simulink model "simulation_pdy_pdx_theta_discreteV2"  (R2015a)
settings: Solver=ode45  StartTime=0.0  StopTime=8000.0  RelTol=1e-3
libraries: simulink x1
settings Model: Creator=MateusVendramini  LastModifiedBy=MateusVendramini
settings SolverCC: AlgebraicLoopSolver=LineSearch

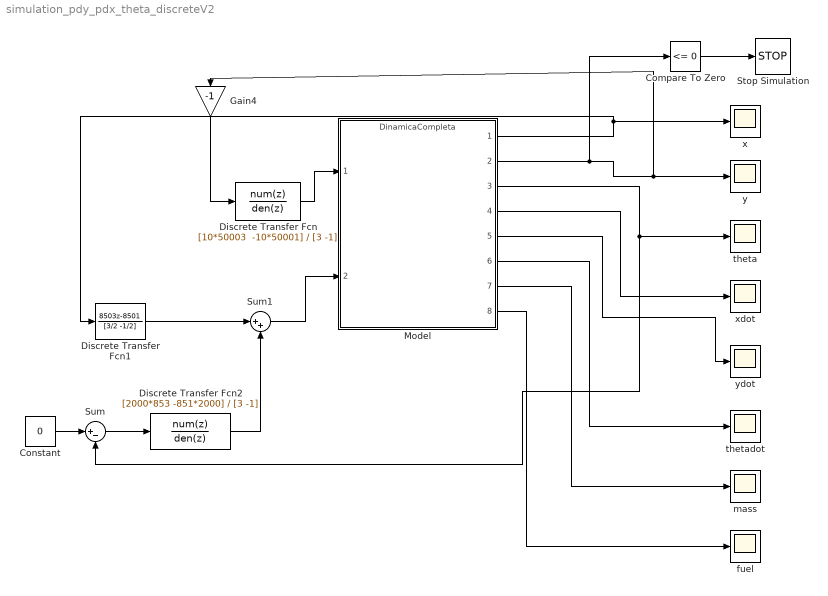
== system simulation_pdy_pdx_theta_discreteV2 ==
  Compare To Zero : simulink/Logic and Bit Operations/Compare To Zero  relop=<=  OutDataTypeStr=boolean
  Constant : Constant  Value=0
  Discrete Transfer Fcn : DiscreteTransferFcn  Numerator="[10*50003  -10*50001]"  Denominator=[3 -1]  SampleTime=0.01
  Discrete Transfer Fcn1 : DiscreteTransferFcn  Numerator=[8503 -8501]  Denominator=[3/2 -1/2]  SampleTime=0.01
  Discrete Transfer Fcn2 : DiscreteTransferFcn  Numerator=[2000*853 -851*2000]  Denominator=[3 -1]  SampleTime=0.01
  Gain4 : Gain  Gain=-1
  Model : ModelReference  ModelNameDialog=DinamicaCompleta.slx  SimulationMode=Normal  ModelReferenceVersion=1.4  CopyOfModelName=DinamicaCompleta.slx  DefaultDataLogging=on
  Stop Simulation : Stop
  Sum : Sum  Inputs=|+-
  Sum1 : Sum  Inputs=|++
  fuel : Scope
      settings: TimeRange=16.32072553815624  YMin=700  YMax=891.0695187165775  SaveName=ScopeData7
  mass : Scope
      settings: SaveName=ScopeData6
  theta : Scope
      settings: SaveName=ScopeData2
  thetadot : Scope
      settings: SaveName=ScopeData5
  x : Scope
      settings: YMin=80  YMax=290
  xdot : Scope
      settings: SaveName=ScopeData3
  y : Scope
      settings: YMin=600000  YMax=2.4e+06  SaveName=Y0001
  ydot : Scope
      settings: SaveName=ScopeData4
  wires:
  Sum/1 -> Discrete Transfer Fcn2/1
  Model/3 -> theta/1, Sum/2
  Model/1 -> Discrete Transfer Fcn1/1, x/1
  Model/2 -> Compare To Zero/1, y/1, Gain4/1
  Model/4 -> xdot/1
  Model/5 -> ydot/1
  Model/6 -> thetadot/1
  Model/7 -> mass/1
  Model/8 -> fuel/1
  Compare To Zero/1 -> Stop Simulation/1
  Discrete Transfer Fcn/1 -> Model/1
  Gain4/1 -> Discrete Transfer Fcn/1
  Discrete Transfer Fcn1/1 -> Sum1/1
  Discrete Transfer Fcn2/1 -> Sum1/2
  Constant/1 -> Sum/1
  Sum1/1 -> Model/2
